simulink model "demo_GS"  (R2023a)
settings: Solver=VariableStepAuto  StartTime=0.0  StopTime=10.0  RelTol=1e-3
values from neighbouring files (symbols this model uses):
  H = 100    [Calculos00_OriginalIgnacio.m]    (also in Calculos02_Vnoladetrim.m; Calculos03_TablaTrimados.m; GenerateDataset_v0.m = vH(j); PI_0_OnlyOneController_V20.m = vH(j))
  slopes = [0, rawslopes(2)]    [PI_6_Tracker_GS.m]    (also in PI_6_Tracker_bigGuy.m)
  TABLEDATA = [1.10335162023 0.00823171458117 -11.0555848055 -0.375153780134 6.18853169798 -34.1001082535 0.0324757076966 -9.89122049893 0.729242255451 -0.683674300952 1.08721495624 0.00509823507416 ... (12710 elements, 2x5x41x31)]    [TableData_002.mat]    (also in TableData_004.mat = [0.174322085341 -0.0514346863342 -0.753716023023 2.529946466; TableData_006.mat = [0.237084016899 -0.0298197541441 -1.42090322153 1.5613882815; TableData_007GS.mat = [0.237084016899 -0.0298197541441 -1.42090322153 1.5613882815; TableData_009.mat = [0.235717817503 -0.0298554739715 -1.40805314109 1.5648466906)
  V = 12    [Calculos00_OriginalIgnacio.m]    (also in Calculos02_Vnoladetrim.m = 6; Calculos03_TablaTrimados.m = vV(k); GenerateDataset_v0.m = vV(i); PI_0_OnlyOneController_V20.m = vV(i))
libraries: simulink_extras x1, simulink x1
settings Model: Creator=ignac  LastModifiedBy=ignac

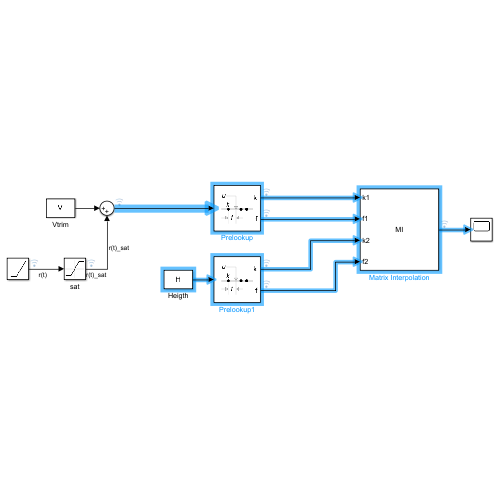
[thumbnail: Simulink's stored preview of the top-level diagram]
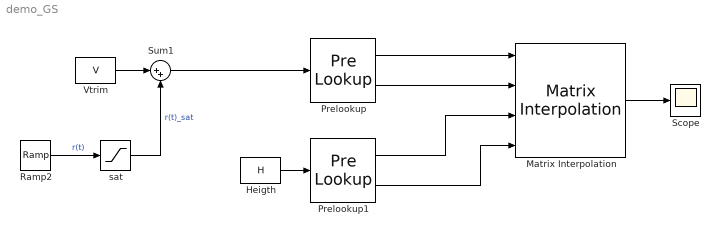
== system demo_GS ==
  Heigth : Constant  Value=H
  Matrix Interpolation : simulink_extras/Additional Lookup Tables/Matrix Interpolation  InterpMethod=Linear  ExtrapMethod=Clip  InterpolateDimension=2  TableData=TABLEDATA  SimulateUsing=Code generation
  Prelookup : PreLookup  BreakpointsData=vV  ExtrapMethod=Linear
  Prelookup1 : PreLookup  BreakpointsData=vH  ExtrapMethod=Linear
  Ramp2 : simulink/Sources/Ramp  slope=slopes  start=0  InitialOutput=0*slopes
  Scope : Scope
  Sum1 : Sum  Inputs=|++
  Vtrim : Constant  Value=V
  sat : Saturate  UpperLimit=slopes*10  LowerLimit=0*slopes
  wires:
  Sum1/1 -> Prelookup/1
  Heigth/1 -> Prelookup1/1
  Vtrim/1 -> Sum1/1
  sat/1 -> Sum1/2  "r(t)_sat"
  Ramp2/1 -> sat/1  "r(t)"
  Prelookup/1 -> Matrix Interpolation/1
  Prelookup/2 -> Matrix Interpolation/2
  Prelookup1/1 -> Matrix Interpolation/3
  Prelookup1/2 -> Matrix Interpolation/4
  Matrix Interpolation/1 -> Scope/1
